simulink model "combinatorial_logic"  (R2020a)
settings: Solver=VariableStepAuto  StartTime=0.0  StopTime=10  RelTol=1e-3
settings Model: Creator=F1  LastModifiedBy=F1

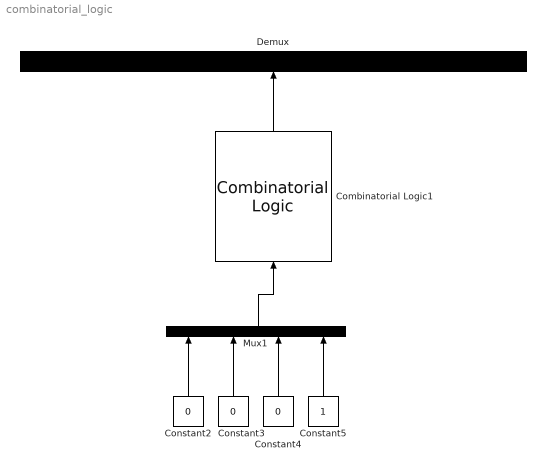
== system combinatorial_logic ==
  Combinatorial Logic1 : CombinatorialLogic  TruthTable=[0 0 0 0 0 1 0 1 0 0;0 0 0 0 1 0 1 0 1 0;0 0 0 0 0 0 0 1 0 1;1 0 0 0 0 0 1 0 0 0;0 0 0 0 0 1 0 1 0 0;0 0 0 0 1 0 1 0 1 0;0 0 0 0 0 0 0 1 0 1;0 0 1 0 0 0 1 0 0 0;0 0 0 0 0 1 0 1 0 0;0 0 0 0 1 0 1 0 1 0;0 0 0 0 0 0 0 0 0 0;0 0 0 0 0 0 0 0 0 0;0 0 0 0 0 1 0 1 0 0; 0 0 0 0 1 0 1 0 1 0;0 0 0 0 0 0 0 0 0 0;0 0 0 0 0 0 0 0 0 0]
  Constant2 : Constant  Value=0  OutDataTypeStr=boolean
  Constant3 : Constant  Value=0  OutDataTypeStr=boolean
  Constant4 : Constant  Value=0  OutDataTypeStr=boolean
  Constant5 : Constant  OutDataTypeStr=boolean
  Demux : Demux  Outputs=10
  Mux1 : Mux
  wires:
  Constant2/1 -> Mux1/1
  Constant3/1 -> Mux1/2
  Mux1/1 -> Combinatorial Logic1/1
  Constant4/1 -> Mux1/3
  Constant5/1 -> Mux1/4
  Combinatorial Logic1/1 -> Demux/1
